simulink model "SyncTime"  (Simulink 9.2)
settings: Solver=ode4  StartTime=1  StopTime=399  FixedStep=.01  RelTol=1e-3  EnableMultiTasking=on
settings Model: Creator=nkymark  LastModifiedBy=markng
settings DebuggingCC: SolverPrmCheckMsg=warning  AllowSymbolicDim=off  StateNameClashWarn=none

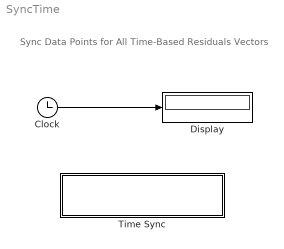
== system SyncTime ==
  note: Sync Data Points for All
      | Time-Based Residuals Vectors
  Clock : Clock
  Display : Display
  "Time Sync " : Subsystem
  wires:
  Clock/1 -> Display/1

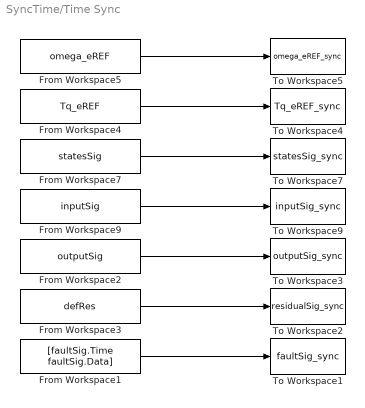
== system SyncTime/Time Sync  ==
  From Workspace1 : FromWorkspace  VariableName=[faultSig.Time faultSig.Data]  SampleTime=0
  From Workspace2 : FromWorkspace  VariableName=outputSig  SampleTime=0
  From Workspace3 : FromWorkspace  VariableName=defRes  SampleTime=0
  From Workspace4 : FromWorkspace  VariableName=Tq_eREF  SampleTime=0
  From Workspace5 : FromWorkspace  VariableName=omega_eREF  SampleTime=0
  From Workspace7 : FromWorkspace  VariableName=statesSig  SampleTime=0
  From Workspace9 : FromWorkspace  VariableName=inputSig  SampleTime=0
  To Workspace1 : ToWorkspace  VariableName=faultSig_sync  SaveFormat=Timeseries  SampleTime=-1
  To Workspace2 : ToWorkspace  VariableName=residualSig_sync  SaveFormat=Timeseries  SampleTime=-1
  To Workspace3 : ToWorkspace  VariableName=outputSig_sync  SaveFormat=Timeseries  SampleTime=-1
  To Workspace4 : ToWorkspace  VariableName=Tq_eREF_sync  SaveFormat=Timeseries  SampleTime=-1
  To Workspace5 : ToWorkspace  VariableName=omega_eREF_sync  SaveFormat=Timeseries  SampleTime=-1
  To Workspace7 : ToWorkspace  VariableName=statesSig_sync  SaveFormat=Timeseries  SampleTime=-1
  To Workspace9 : ToWorkspace  VariableName=inputSig_sync  SaveFormat=Timeseries  SampleTime=-1
  wires:
  From Workspace9/1 -> To Workspace9/1
  From Workspace3/1 -> To Workspace2/1
  From Workspace1/1 -> To Workspace1/1
  From Workspace2/1 -> To Workspace3/1
  From Workspace4/1 -> To Workspace4/1
  From Workspace5/1 -> To Workspace5/1
  From Workspace7/1 -> To Workspace7/1
